simulink model "questao9"  (R2023a)
settings: Solver=VariableStepAuto  StartTime=0.0  StopTime=250  FixedStep=1  MaxStep=0.1  RelTol=1e-3
values from neighbouring files (symbols this model uses):
  B = 0.1    [trab_controle.m]
  J = 1    [trab_controle.m]
  Km = 1/3    (= 0.333333333333)    [trab_controle.m]
  L = 0.5    [trab_controle.m]
  R = 10    [trab_controle.m]
settings Model: Creator=franz  LastModifiedBy=franz

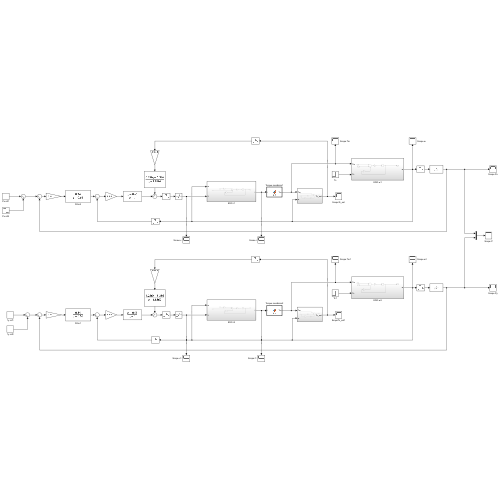
[thumbnail: Simulink's stored preview of the top-level diagram]
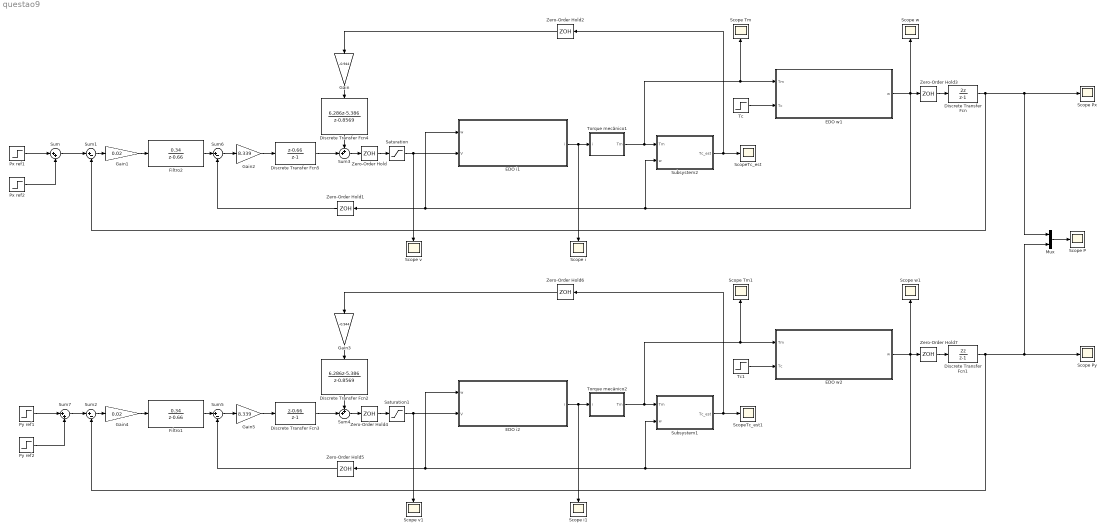
== system questao9 ==
  Discrete Transfer Fcn : DiscreteTransferFcn  Numerator=[2 0]  Denominator=[1 -1]
  Discrete Transfer Fcn1 : DiscreteTransferFcn  Numerator=[2 0]  Denominator=[1 -1]
  Discrete Transfer Fcn2 : DiscreteTransferFcn  Numerator=[6.286 -5.386]  Denominator=[1 -0.8569]
  Discrete Transfer Fcn3 : DiscreteTransferFcn  Numerator=[1 -0.66]  Denominator=[1 -1]
  Discrete Transfer Fcn4 : DiscreteTransferFcn  Numerator=[6.286 -5.386]  Denominator=[1 -0.8569]
  Discrete Transfer Fcn5 : DiscreteTransferFcn  Numerator=[1 -0.66]  Denominator=[1 -1]
  EDO i1 : Subsystem
  EDO i2 : Subsystem
  EDO w1 : Subsystem
  EDO w2 : Subsystem
  Filtro1 : DiscreteTransferFcn  Numerator=[0 0.34]  Denominator=[1 -0.66]
  Filtro2 : DiscreteTransferFcn  Numerator=[0 0.34]  Denominator=[1 -0.66]
  Gain : Gain  Gain=-0.944
  Gain1 : Gain  Gain=0.02
  Gain2 : Gain  Gain=8.339
  Gain3 : Gain  Gain=-0.944
  Gain4 : Gain  Gain=0.02
  Gain5 : Gain  Gain=8.339
  Mux : Mux  Inputs=2
  Px ref1 : Step  Time=120  After=5  SampleTime=0
  Px ref2 : Step  Time=200  After=-5  SampleTime=0
  Py ref1 : Step  Time=80  After=5  SampleTime=0
  Py ref2 : Step  Time=160  After=-5  SampleTime=0
  Saturation : Saturate  UpperLimit=40  LowerLimit=-40
  Saturation1 : Saturate  UpperLimit=40  LowerLimit=-40
  Scope P : Scope
  Scope Px : Scope
  Scope Py : Scope
  Scope Tm : Scope
  Scope Tm1 : Scope
  Scope i : Scope
  Scope i1 : Scope
  Scope v : Scope
  Scope v1 : Scope
  Scope w : Scope
  Scope w1 : Scope
  ScopeTc_est : Scope
  ScopeTc_est1 : Scope
  Subsystem1 : Subsystem
  Subsystem2 : Subsystem
  Sum : Sum  Inputs=|++
  Sum{1..2,5..6} (4 alike) : Sum  Inputs=|+-
  Sum3 : Sum  Inputs=++|
  Sum4 : Sum  Inputs=++|
  Sum7 : Sum  Inputs=|++
  Tc : Step  Time=120  Before=2  After=2  SampleTime=0
  Tc1 : Step  Time=120  Before=2  After=2  SampleTime=0
  Torque mecânico1 : MATLAB Function  TreatAsAtomicUnit=on
  Torque mecânico2 : MATLAB Function  TreatAsAtomicUnit=on
  Zero-Order Hold{,1..7} (8 alike) : ZeroOrderHold  SampleTime=-1
  wires:
  Discrete Transfer Fcn5/1 -> Sum3/2
  Filtro2/1 -> Sum6/1
  Discrete Transfer Fcn4/1 -> Sum3/1
  Sum6/1 -> Gain2/1
  Gain2/1 -> Discrete Transfer Fcn5/1
  Subsystem2/1(Tc_est) -> ScopeTc_est/1, Zero-Order Hold2/1
  EDO i1/1(i) -> Torque mecânico1/1(i), Scope i/1
  Torque mecânico1/1(Tm) -> Subsystem2/1(Tm), EDO w1/1(Tm), Scope Tm/1
  Tc/1 -> EDO w1/2(Tc)
  EDO w1/1(w) -> Zero-Order Hold3/1, Zero-Order Hold1/1, EDO i1/1(w), Subsystem2/2(w), Scope w/1
  Sum3/1 -> Zero-Order Hold/1
  Gain/1 -> Discrete Transfer Fcn4/1
  Zero-Order Hold/1 -> Saturation/1
  Zero-Order Hold1/1 -> Sum6/2
  Zero-Order Hold2/1 -> Gain/1
  Saturation/1 -> EDO i1/2(V), Scope v/1
  Discrete Transfer Fcn/1 -> Mux/1, Scope Px/1, Sum1/2
  Sum1/1 -> Gain1/1
  Gain1/1 -> Filtro2/1
  Zero-Order Hold3/1 -> Discrete Transfer Fcn/1
  Sum7/1 -> Sum2/1
  Subsystem1/1(Tc_est) -> ScopeTc_est1/1, Zero-Order Hold6/1
  Zero-Order Hold7/1 -> Discrete Transfer Fcn1/1
  Saturation1/1 -> EDO i2/2(V), Scope v1/1
  Tc1/1 -> EDO w2/2(Tc)
  Zero-Order Hold6/1 -> Gain3/1
  Torque mecânico2/1(Tm) -> Subsystem1/1(Tm), EDO w2/1(Tm), Scope Tm1/1
  Sum4/1 -> Zero-Order Hold4/1
  Gain4/1 -> Filtro1/1
  Sum2/1 -> Gain4/1
  Zero-Order Hold5/1 -> Sum5/2
  Discrete Transfer Fcn1/1 -> Mux/2, Scope Py/1, Sum2/2
  EDO w2/1(w) -> Zero-Order Hold7/1, Zero-Order Hold5/1, EDO i2/1(w), Subsystem1/2(w), Scope w1/1
  Gain3/1 -> Discrete Transfer Fcn2/1
  Zero-Order Hold4/1 -> Saturation1/1
  Sum5/1 -> Gain5/1
  EDO i2/1(i) -> Torque mecânico2/1(i), Scope i1/1
  Filtro1/1 -> Sum5/1
  Discrete Transfer Fcn3/1 -> Sum4/2
  Gain5/1 -> Discrete Transfer Fcn3/1
  Discrete Transfer Fcn2/1 -> Sum4/1
  Px ref1/1 -> Sum/1
  Px ref2/1 -> Sum/2
  Sum/1 -> Sum1/1
  Py ref2/1 -> Sum7/2
  Py ref1/1 -> Sum7/1
  Mux/1 -> Scope P/1

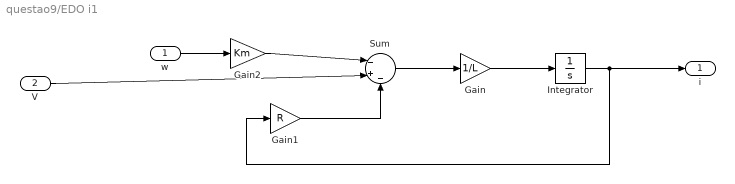
== system questao9/EDO i1 ==
  w : Inport
  V : Inport  Port=2
  Gain : Gain  Gain=1/L
  Gain1 : Gain  Gain=R
  Gain2 : Gain  Gain=Km
  Integrator : Integrator
  Sum : Sum  Inputs=|-+-
  i : Outport
  wires:
  Gain1/1 -> Sum/3
  Integrator/1 -> i/1, Gain1/1
  Gain/1 -> Integrator/1
  Sum/1 -> Gain/1
  w/1 -> Gain2/1
  Gain2/1 -> Sum/1
  V/1 -> Sum/2

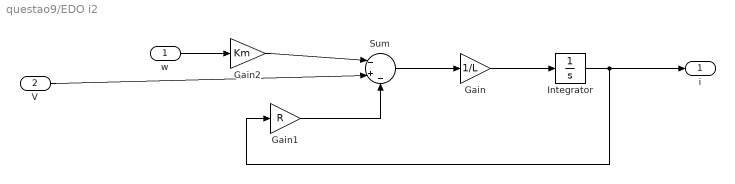
== system questao9/EDO i2 ==
  w : Inport
  V : Inport  Port=2
  Gain : Gain  Gain=1/L
  Gain1 : Gain  Gain=R
  Gain2 : Gain  Gain=Km
  Integrator : Integrator
  Sum : Sum  Inputs=|-+-
  i : Outport
  wires:
  Gain1/1 -> Sum/3
  Integrator/1 -> i/1, Gain1/1
  Gain/1 -> Integrator/1
  Sum/1 -> Gain/1
  w/1 -> Gain2/1
  Gain2/1 -> Sum/1
  V/1 -> Sum/2

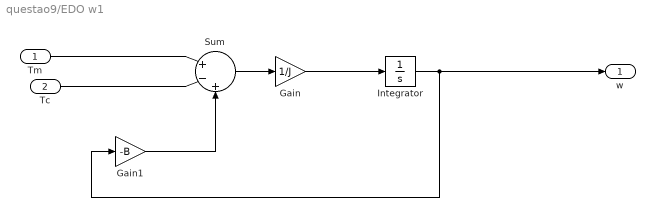
== system questao9/EDO w1 ==
  Tm : Inport
  Tc : Inport  Port=2
  Gain : Gain  Gain=1/J
  Gain1 : Gain  Gain=-B
  Integrator : Integrator
  Sum : Sum  Inputs=|+-+
  w : Outport
  wires:
  Tm/1 -> Sum/1
  Sum/1 -> Gain/1
  Tc/1 -> Sum/2
  Gain/1 -> Integrator/1
  Gain1/1 -> Sum/3
  Integrator/1 -> Gain1/1, w/1

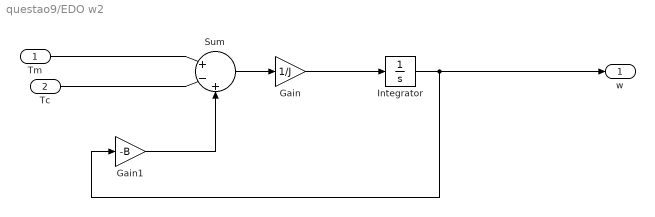
== system questao9/EDO w2 ==
  Tm : Inport
  Tc : Inport  Port=2
  Gain : Gain  Gain=1/J
  Gain1 : Gain  Gain=-B
  Integrator : Integrator
  Sum : Sum  Inputs=|+-+
  w : Outport
  wires:
  Tm/1 -> Sum/1
  Sum/1 -> Gain/1
  Tc/1 -> Sum/2
  Gain/1 -> Integrator/1
  Gain1/1 -> Sum/3
  Integrator/1 -> Gain1/1, w/1

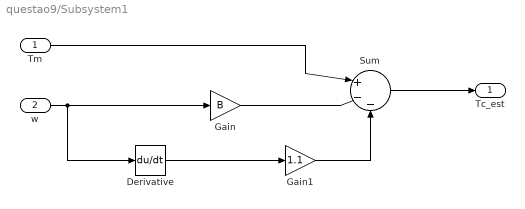
== system questao9/Subsystem1 ==
  Tm : Inport
  w : Inport  Port=2
  Derivative : Derivative
  Gain : Gain  Gain=B
  Gain1 : Gain  Gain=1.1
  Sum : Sum  Inputs=|+--
  Tc_est : Outport
  wires:
  w/1 -> Derivative/1, Gain/1
  Gain/1 -> Sum/2
  Tm/1 -> Sum/1
  Derivative/1 -> Gain1/1
  Gain1/1 -> Sum/3
  Sum/1 -> Tc_est/1

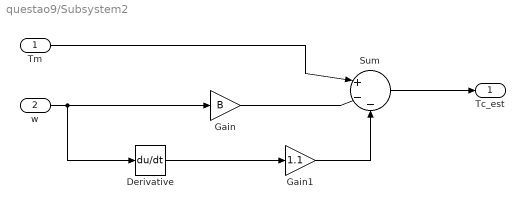
== system questao9/Subsystem2 ==
  Tm : Inport
  w : Inport  Port=2
  Derivative : Derivative
  Gain : Gain  Gain=B
  Gain1 : Gain  Gain=1.1
  Sum : Sum  Inputs=|+--
  Tc_est : Outport
  wires:
  w/1 -> Derivative/1, Gain/1
  Gain/1 -> Sum/2
  Tm/1 -> Sum/1
  Derivative/1 -> Gain1/1
  Gain1/1 -> Sum/3
  Sum/1 -> Tc_est/1

== matlab function questao9/Torque mecânico1 ==
  data: i input; Tm output
function Tm = fcn(i)

if i >= 0
    torque_m = 5.26*(1 - exp(-i));
else
    torque_m = -5.26*(1 - exp(i));
end
Tm = torque_m;

== matlab function questao9/Torque mecânico2 ==
  data: i input; Tm output
function Tm = fcn(i)

if i >= 0
    torque_m = 5.26*(1 - exp(-i));
else
    torque_m = -5.26*(1 - exp(i));
end
Tm = torque_m;
